simulink model "KITTRacing"  (R2017a)
settings: Solver=FixedStepAuto  StartTime=0.0  StopTime=5  FixedStep=0.01  RelTol=1e-3
values from neighbouring files (symbols this model uses):
  b = 0.0015    [KITTParameters.m]    (also in MakeBrakingCurve.m = 18.5)
  c = 0.02    [KITTParameters.m]    (also in MakeAccelerationCurve.m = 0)
  Fa = 0    [KITTDynamicsfinal.m]
  Fb = Fb_max    [KITTDynamicsfinal.m]
  m = 13    [KITTParameters.m]
  v0 = 40    [KITTDynamicsfinal.m]    (also in KITTParameters.m = 0)
settings Model: Creator=Robert  LastModifiedBy=Robert
settings DataIOCC: LimitDataPoints=on  SaveOutput=off  SaveTime=off
settings OptimizationCC: BlockReduction=off  BooleanDataType=off  LifeSpan=inf
settings DebuggingCC: SaveWithParameterizedLinksMsg=none  UnderspecifiedInitializationDetection=Classic  MergeDetectMultiDrivingBlocksExec=none  SignalResolutionControl=TryResolveAllWithWarning  AllowSymbolicDim=off  SFUnexpectedBacktrackingDiag=warning  SFNoUnconditionalDefaultTransitionDiag=warning  SFExecutionAtInitializationDiag=none
settings HardwareCC: TargetUnknown=on
settings GRTTargetCC: TargetLangStandard=C89/C90 (ANSI)  GeneratePreprocessorConditionals=Disable all

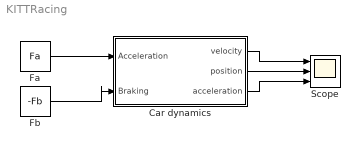
== system KITTRacing ==
  Car dynamics : Subsystem
  Fa : Constant  Value=Fa
  Fb : Constant  Value=-Fb
  Scope : Scope  NumInputPorts=3
  wires:
  Fa/1 -> Car dynamics/1(Acceleration)
  Fb/1 -> Car dynamics/2(Braking)
  Car dynamics/1(velocity) -> Scope/1
  Car dynamics/2(position) -> Scope/2
  Car dynamics/3(acceleration) -> Scope/3

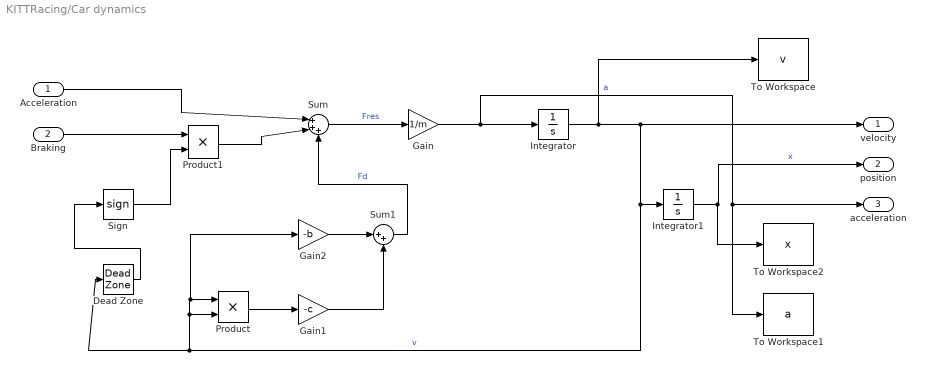
== system KITTRacing/Car dynamics ==
  Acceleration : Inport
  Braking : Inport  Port=2
  Dead Zone : DeadZone  LowerValue=-0.1  UpperValue=0.1  SaturateOnIntegerOverflow=on
  Gain : Gain  Gain=1/m
  Gain1 : Gain  Gain=-c
  Gain2 : Gain  Gain=-b
  Integrator : Integrator  InitialCondition=v0
  Integrator1 : Integrator
  Product : Product
  Product1 : Product
  Sign : Signum
  Sum : Sum  Inputs=|+++
  Sum1 : Sum  Inputs=|++
  To Workspace : ToWorkspace  VariableName=v  SaveFormat=Structure With Time  SampleTime=-1
      settings: Save2DSignal=2-D array (concatenate along first dimension)
  To Workspace1 : ToWorkspace  VariableName=a  SaveFormat=Structure With Time  SampleTime=-1
      settings: Save2DSignal=2-D array (concatenate along first dimension)
  To Workspace2 : ToWorkspace  VariableName=x  SaveFormat=Structure With Time  SampleTime=-1
      settings: Save2DSignal=2-D array (concatenate along first dimension)
  velocity : Outport
  position : Outport  Port=2
  acceleration : Outport  Port=3
  wires:
  Acceleration/1 -> Sum/1
  Product/1 -> Gain1/1
  Braking/1 -> Product1/1
  Gain/1 -> To Workspace1/1, acceleration/1, Integrator/1  "a"
  Sum1/1 -> Sum/3  "Fd"
  Sign/1 -> Product1/2
  Dead Zone/1 -> Sign/1
  Product1/1 -> Sum/2
  Integrator/1 -> velocity/1, Integrator1/1, Dead Zone/1, Gain2/1, Product/1, Product/2, To Workspace/1  "v"
  Sum/1 -> Gain/1  "Fres"
  Gain1/1 -> Sum1/2
  Integrator1/1 -> To Workspace2/1, position/1  "x"
  Gain2/1 -> Sum1/1
